simulink model "Ex5_3"  (R2016b)
settings: Solver=VariableStepAuto  StartTime=0.0  StopTime=runtime  RelTol=1e-3
values from neighbouring files (symbols this model uses):
  g = 9.81    [Ex5_3_init.m]
  i_smn0 = zeros(2,1)    [Ex5_3_init.m]
  J = 0.05    [Ex5_2_init.m]    (also in Ex5_3_init.m; Home54_init.m = 0.5; homepart51.m)
  Kd = 1    [Ex5_3_init.m]
  Ki = 1    [Ex5_3_init.m]
  Kp = 120    [Ex5_3_init.m]
  L_s = 0.085    [Ex5_2_init.m]    (also in Ex5_3_init.m; Home54_init.m)
  m = 40    [Ex5_3_init.m]
  p = 1    [Ex5_2_init.m]    (also in Ex5_3_init.m; Home54_init.m; homepart51.m)
  psi_Rmn0 = zeros(2,1)    [Ex5_3_init.m]
  r = 0.1    [Ex5_3_init.m]
  sigma = 1 - M^2/(L_s*L_r)    (= 0.0693425605536)    [Ex5_2_init.m]    (also in Ex5_3_init.m = 0.0693; Home54_init.m = 0.0693; homepart51.m)
  tau_r = 0.283    [Ex5_3_init.m]    (also in Home54_init.m)
  tau_sigma = 0.0102    [Ex5_3_init.m]
  U0 = 22    [Ex5_3_init.m]
  Us = sqrt(2)*Uphase    [Ex5_2_init.m]    (also in Ex5_3_init.m = Us_rat/Ws_rat * ws)
  Us_rat = Us    [Ex5_3_init.m]
  Wk = 50*2*pi    (= 314.159265359)    [Ex5_3_init.m]
  ws = 50*2*pi    (= 314.159265359)    [Ex5_2_init.m]    (also in Ex5_3_init.m)
  Ws_rat = 50*2*pi    (= 314.159265359)    [Ex5_3_init.m]
  Wslip_max = 49    [Ex5_3_init.m]
undefined symbols (not defined in the file or in its folder): sigbuilder_block
settings Model: Creator=Niels  LastModifiedBy=Niels

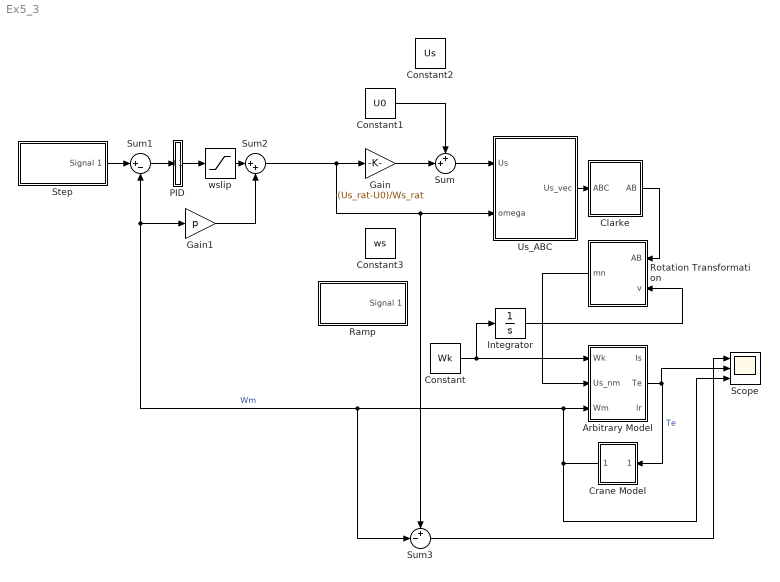
== system Ex5_3 ==
  Arbitrary Model : Subsystem
  Clarke : Subsystem
  Constant : Constant  Value=Wk
  Constant1 : Constant  Value=U0
  Constant2 : Constant  Value=Us
  Constant3 : Constant  Value=ws
  Crane Model : Subsystem
  Gain : Gain  Gain=(Us_rat-U0)/Ws_rat
  Gain1 : Gain  Gain=p
  Integrator : Integrator
  PID : Subsystem
  Ramp : Subsystem  Tag=STV Subsys  LoadFcn=sigbuilder_block('load');  StartFcn=sigbuilder_block('start');  StopFcn=sigbuilder_block('stop');  ClipboardFcn=sigbuilder_block('clipboard');  mask(Sigbuilder block){tuvar=[0:10]}
      mask help: Simulink:masks:SigbuilderBlock_MD
      mask init:
      | if ~strcmp(get_param(bdroot(gcbh),'SimulationStatus'),'stopped') tuvar = sigbuilder_block('maskInit'); end
      settings: CopyFcn=sigbuilder_block('copy');  DeleteFcn=sigbuilder_block('delete');  ModelCloseFcn=sigbuilder_block('modelClose');  PreSaveFcn=sigbuilder_block('preSave');  PauseFcn=sigbuilder_block('pause');  ContinueFcn=sigbuilder_block('continue');  NameChangeFcn=sigbuilder_block('namechange');  OpenFcn=sigbuilder_block('open',[437.6 199.2 550.4 400 ]);  CloseFcn=sigbuilder_block('close');
      mask Display: plot(0, 0, 100, 100,[2, 2, 32, 32, 2], [68, 8, 8, 68, 68],[32, 2], [38, 38], [32, 19, 2],[53, 60, 44], [32, 17, 17, 2],[16, 16, 31, 31]);txt = getActiveGroup(gcbh);text(2, 100, txt,'verticalAlignment', 'top');
  "Rotation Transformation " : Subsystem
  Scope : Scope  NumInputPorts=3
  Step : Subsystem  Tag=STV Subsys  LoadFcn=sigbuilder_block('load');  StartFcn=sigbuilder_block('start');  StopFcn=sigbuilder_block('stop');  ClipboardFcn=sigbuilder_block('clipboard');  mask(Sigbuilder block){tuvar=[0:10]}
      mask help: Simulink:masks:SigbuilderBlock_MD
      mask init:
      | if ~strcmp(get_param(bdroot(gcbh),'SimulationStatus'),'stopped') tuvar = sigbuilder_block('maskInit'); end
      settings: CopyFcn=sigbuilder_block('copy');  DeleteFcn=sigbuilder_block('delete');  ModelCloseFcn=sigbuilder_block('modelClose');  PreSaveFcn=sigbuilder_block('preSave');  PauseFcn=sigbuilder_block('pause');  ContinueFcn=sigbuilder_block('continue');  NameChangeFcn=sigbuilder_block('namechange');  OpenFcn=sigbuilder_block('open',[437.6 199.2 550.4 400 ]);  CloseFcn=sigbuilder_block('close');
      mask Display: plot(0, 0, 100, 100,[2, 2, 32, 32, 2], [68, 8, 8, 68, 68],[32, 2], [38, 38], [32, 19, 2],[53, 60, 44], [32, 17, 17, 2],[16, 16, 31, 31]);txt = getActiveGroup(gcbh);text(2, 100, txt,'verticalAlignment', 'top');
  Sum : Sum  Inputs=++|
  Sum1 : Sum  Inputs=|+-
  Sum2 : Sum  Inputs=|++
  Sum3 : Sum  Inputs=+-|
  Us_ABC : Subsystem
  wslip : Saturate  UpperLimit=Wslip_max  LowerLimit=-Wslip_max
  wires:
  Us_ABC/1(Us_vec) -> Clarke/1(ABC)
  Arbitrary Model/2(Te) -> Scope/2, Crane Model/1(Te)  "Te"
  Crane Model/1(wm) -> Scope/3, Arbitrary Model/3(Wm), Sum3/2, Gain1/1, Sum1/2  "Wm"
  Clarke/1(AB) -> "Rotation Transformation "/1(AB)
  "Rotation Transformation "/1(mn) -> Arbitrary Model/2(Us_nm)
  Integrator/1 -> "Rotation Transformation "/2(v)
  Gain/1 -> Sum/2
  Constant1/1 -> Sum/1
  Constant/1 -> Arbitrary Model/1(Wk), Integrator/1
  Step/1(Signal 1) -> Sum1/1
  Sum1/1 -> PID/1(In1)
  wslip/1 -> Sum2/1
  Sum2/1 -> Us_ABC/2(omega), Sum3/1, Gain/1
  Gain1/1 -> Sum2/2
  PID/1(Out1) -> wslip/1
  Sum3/1 -> Scope/1
  Sum/1 -> Us_ABC/1(Us)

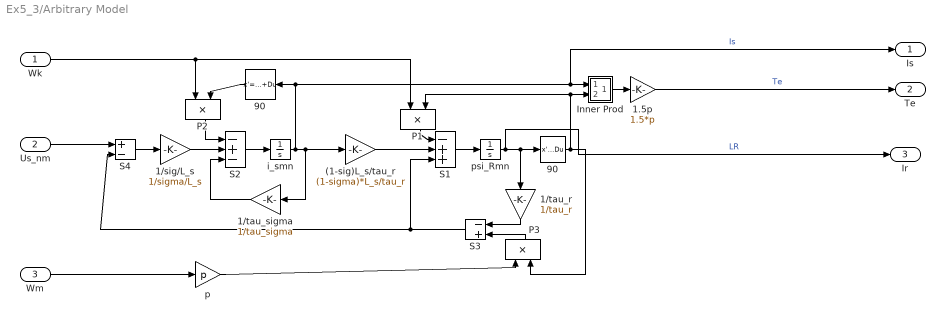
== system Ex5_3/Arbitrary Model ==
  Wk : Inport
  Us_nm : Inport  Port=2
  Wm : Inport  Port=3
  (1-sig)L_s/tau_r : Gain  Gain=(1-sigma)*L_s/tau_r  SaturateOnIntegerOverflow=on  OutDataTypeStr=Inherit: Same as input  ParamDataTypeStr=Inherit: Same as input
  1.5p : Gain  Gain=1.5*p  SaturateOnIntegerOverflow=on  OutDataTypeStr=Inherit: Same as input  ParamDataTypeStr=Inherit: Same as input
  1/sig/L_s : Gain  Gain=1/sigma/L_s  SaturateOnIntegerOverflow=on  OutDataTypeStr=Inherit: Same as input  ParamDataTypeStr=Inherit: Same as input
  1/tau_r : Gain  Gain=1/tau_r  SaturateOnIntegerOverflow=on  OutDataTypeStr=Inherit: Same as input  ParamDataTypeStr=Inherit: Same as input
  1/tau_sigma : Gain  Gain=1/tau_sigma  SaturateOnIntegerOverflow=on  OutDataTypeStr=Inherit: Same as input  ParamDataTypeStr=Inherit: Same as input
  90 : StateSpace  A=[]  B=[]  C=[]  D=K  X0=0  mask(Matrix gain){K=[0 -1;1 0]}
      mask prompts: K "Gain matrix:"
      mask help: Matrix Gain.
      mask Help: Multiplies input vector by entered matrix to produce output vector (y=Au).
      mask Display: disp('K')
  "90 " : StateSpace  A=[]  B=[]  C=[]  D=K  X0=0  mask(Matrix gain){K=[0 -1;1 0]}
      mask prompts: K "Gain matrix:"
      mask help: Matrix Gain.
      mask Help: Multiplies input vector by entered matrix to produce output vector (y=Au).
      mask Display: disp('K')
  Inner Prod : Subsystem  mask(Dot Product){}
      mask help:
      | Inner (dot) product.
      | y=sum(u1.*u2)
      mask Help: Computes the inner (dot) product of the inputs: sum(u1.*u2).  The inputs are vectors of the same length. Output is a scalar.
      mask Display: disp('.\n')
  P1 : Product  SaturateOnIntegerOverflow=on  RndMeth=Zero  InputSameDT=on  OutDataTypeStr=Inherit: Same as first input
  P2 : Product  SaturateOnIntegerOverflow=on  RndMeth=Zero  InputSameDT=on  OutDataTypeStr=Inherit: Same as first input
  P3 : Product  SaturateOnIntegerOverflow=on  RndMeth=Zero  InputSameDT=on  OutDataTypeStr=Inherit: Same as first input
  S1 : Sum  Inputs=-++  SaturateOnIntegerOverflow=on  InputSameDT=on  OutDataTypeStr=Inherit: Same as first input
  S2 : Sum  Inputs=-+-  SaturateOnIntegerOverflow=on  InputSameDT=on  OutDataTypeStr=Inherit: Same as first input
  S3 : Sum  Inputs=-+  SaturateOnIntegerOverflow=on  InputSameDT=on  OutDataTypeStr=Inherit: Same as first input
  S4 : Sum  Inputs=+-  SaturateOnIntegerOverflow=on  InputSameDT=on  OutDataTypeStr=Inherit: Same as first input
  i_smn : Integrator  InitialCondition=i_smn0
  "p " : Gain  Gain=p  SaturateOnIntegerOverflow=on  OutDataTypeStr=Inherit: Same as input  ParamDataTypeStr=Inherit: Same as input
  psi_Rmn : Integrator  InitialCondition=psi_Rmn0
  Is : Outport
  Te : Outport  Port=2
  Ir : Outport  Port=3
  wires:
  P2/1 -> S2/1
  Wm/1 -> "p "/1
  S4/1 -> 1/sig/L_s/1
  "p "/1 -> P3/1
  "90 "/1 -> P3/2, Inner Prod/2(in_2), P1/2
  S3/1 -> S1/3, S4/2
  S2/1 -> i_smn/1
  1/tau_sigma/1 -> S2/3
  P1/1 -> S1/1
  (1-sig)L_s/tau_r/1 -> S1/2
  1.5p/1 -> Te/1  "Te"
  Us_nm/1 -> S4/1
  1/tau_r/1 -> S3/1
  S1/1 -> psi_Rmn/1
  Inner Prod/1(out_1) -> 1.5p/1
  psi_Rmn/1 -> Ir/1, "90 "/1, 1/tau_r/1  "LR"
  P3/1 -> S3/2
  Wk/1 -> P1/1, P2/1
  90/1 -> P2/2
  i_smn/1 -> (1-sig)L_s/tau_r/1, 1/tau_sigma/1, 90/1, Is/1, Inner Prod/1(in_1)  "Is"
  1/sig/L_s/1 -> S2/2

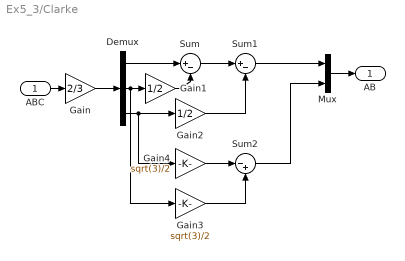
== system Ex5_3/Clarke ==
  ABC : Inport
  Demux : Demux  Outputs=3
  Gain : Gain  Gain=2/3
  Gain1 : Gain  Gain=1/2
  Gain2 : Gain  Gain=1/2
  Gain3 : Gain  Gain=sqrt(3)/2
  Gain4 : Gain  Gain=sqrt(3)/2
  Mux : Mux  Inputs=2
  Sum : Sum  Inputs=|+-
  Sum1 : Sum  Inputs=|+-
  Sum2 : Sum  Inputs=|-+
  AB : Outport
  wires:
  ABC/1 -> Gain/1
  Mux/1 -> AB/1
  Gain/1 -> Demux/1
  Demux/1 -> Sum/1
  Demux/2 -> Gain3/1, Gain1/1
  Gain1/1 -> Sum/2
  Sum/1 -> Sum1/1
  Sum1/1 -> Mux/1
  Demux/3 -> Gain4/1, Gain2/1
  Gain2/1 -> Sum1/2
  Gain4/1 -> Sum2/1
  Gain3/1 -> Sum2/2
  Sum2/1 -> Mux/2

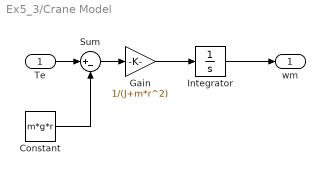
== system Ex5_3/Crane Model ==
  Te : Inport
  Constant : Constant  Value=m*g*r
  Gain : Gain  Gain=1/(J+m*r^2)
  Integrator : Integrator
  Sum : Sum  Inputs=|+-
  wm : Outport
  wires:
  Gain/1 -> Integrator/1
  Integrator/1 -> wm/1
  Te/1 -> Sum/1
  Sum/1 -> Gain/1
  Constant/1 -> Sum/2

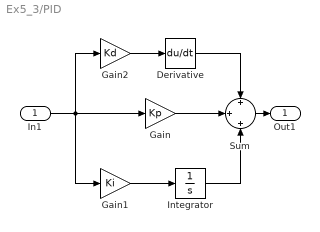
== system Ex5_3/PID ==
  In1 : Inport
  Derivative : Derivative
  Gain : Gain  Gain=Kp
  Gain1 : Gain  Gain=Ki
  Gain2 : Gain  Gain=Kd
  Integrator : Integrator
  Sum : Sum  Inputs=+|+|+
  Out1 : Outport
  wires:
  In1/1 -> Gain2/1, Gain1/1, Gain/1
  Gain1/1 -> Integrator/1
  Sum/1 -> Out1/1
  Gain/1 -> Sum/2
  Integrator/1 -> Sum/3
  Gain2/1 -> Derivative/1
  Derivative/1 -> Sum/1

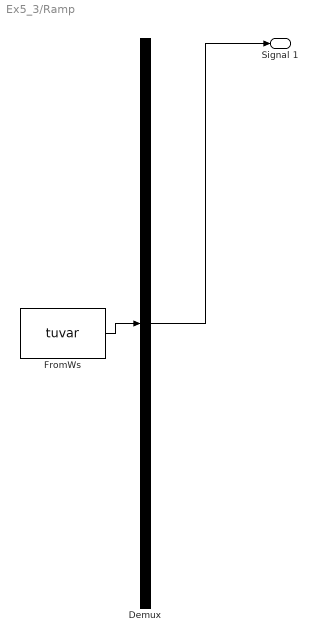
== system Ex5_3/Ramp ==
  Demux : Demux  Tag=STV Demux  Outputs=1
  FromWs : FromWorkspace  Tag=STV FromWs  VariableName=tuvar  SampleTime=0
      SigBuilderData=|
      | common.afterFinalStr = 'Extrapolate'
      | common.sampleTime = 0
      | dataSet.timeRange = [0 100]
      | dataSet.name = 'Group 1'
      | sbobj.Groups.Name = 'Group 1'
      | sbobj.Groups.Signals.Name = 'Signal 1'
      | sbobj.Groups.Signals.XData = [0 3 100]
      | sbobj.Groups.Signals.YData = [56.5486677646 314.159265359 314.159265359]
      | sbobj.Groups.TimeRange = [0 100]
  Signal 1 : Outport  Tag=STV Outport
  wires:
  Demux/1 -> Signal 1/1
  FromWs/1 -> Demux/1

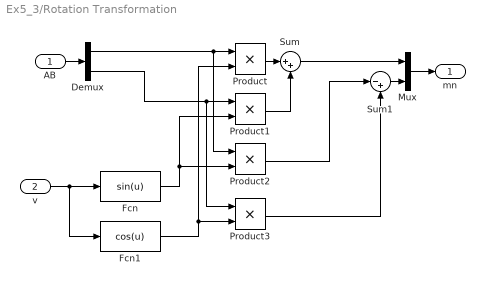
== system Ex5_3/Rotation Transformation  ==
  AB : Inport
  v : Inport  Port=2
  Demux : Demux  Outputs=2
  Fcn : Fcn  Expr=sin(u)
  Fcn1 : Fcn  Expr=cos(u)
  Mux : Mux  Inputs=2
  Product{,1..3} (4 alike) : Product
  Sum : Sum  Inputs=|++
  Sum1 : Sum  Inputs=|-+
  mn : Outport
  wires:
  v/1 -> Fcn1/1, Fcn/1
  Mux/1 -> mn/1
  AB/1 -> Demux/1
  Sum/1 -> Mux/1
  Product/1 -> Sum/1
  Demux/1 -> Product2/1, Product/1
  Fcn1/1 -> Product3/2, Product/2
  Demux/2 -> Product3/1, Product1/1
  Fcn/1 -> Product2/2, Product1/2
  Product1/1 -> Sum/2
  Sum1/1 -> Mux/2
  Product2/1 -> Sum1/1
  Product3/1 -> Sum1/2

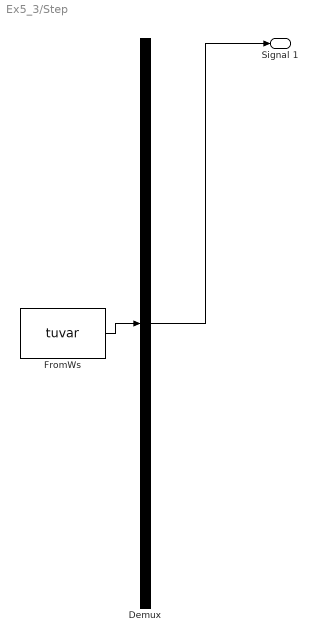
== system Ex5_3/Step ==
  Demux : Demux  Tag=STV Demux  Outputs=1
  FromWs : FromWorkspace  Tag=STV FromWs  VariableName=tuvar  SampleTime=0
      SigBuilderData=|
      | common.afterFinalStr = 'Extrapolate'
      | common.sampleTime = 0
      | dataSet.timeRange = [0 10]
      | dataSet.name = 'Group 1'
      | sbobj.Groups.Name = 'Group 1'
      | sbobj.Groups.Signals.Name = 'Signal 1'
      | sbobj.Groups.Signals.XData = [0 10]
      | sbobj.Groups.Signals.YData = [314.159265359 314.159265359]
  Signal 1 : Outport  Tag=STV Outport
  wires:
  Demux/1 -> Signal 1/1
  FromWs/1 -> Demux/1

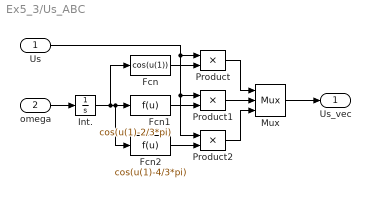
== system Ex5_3/Us_ABC ==
  Us : Inport
  omega : Inport  Port=2
  Fcn : Fcn  Expr=cos(u(1))
  Fcn1 : Fcn  Expr=cos(u(1)-2/3*pi)
  Fcn2 : Fcn  Expr=cos(u(1)-4/3*pi)
  Int. : Integrator
  Mux : Mux  Inputs=3
  Product : Product  SaturateOnIntegerOverflow=on  RndMeth=Zero  InputSameDT=on  OutDataTypeStr=Inherit: Same as first input
  Product1 : Product  SaturateOnIntegerOverflow=on  RndMeth=Zero  InputSameDT=on  OutDataTypeStr=Inherit: Same as first input
  Product2 : Product  SaturateOnIntegerOverflow=on  RndMeth=Zero  InputSameDT=on  OutDataTypeStr=Inherit: Same as first input
  Us_vec : Outport
  wires:
  Fcn2/1 -> Product2/2
  Fcn1/1 -> Product1/2
  Product/1 -> Mux/1
  Product2/1 -> Mux/3
  Mux/1 -> Us_vec/1
  Product1/1 -> Mux/2
  omega/1 -> Int./1
  Us/1 -> Product/1, Product1/1, Product2/1
  Fcn/1 -> Product/2
  Int./1 -> Fcn1/1, Fcn2/1, Fcn/1

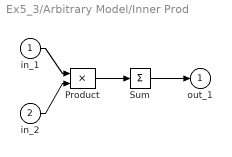
== system Ex5_3/Arbitrary Model/Inner Prod ==
  in_1 : Inport
  in_2 : Inport  Port=2
  Product : Product  SaturateOnIntegerOverflow=on  RndMeth=Zero  InputSameDT=on  OutDataTypeStr=Inherit: Same as first input
  Sum : Sum  Inputs=+  SaturateOnIntegerOverflow=on  InputSameDT=on  OutDataTypeStr=Inherit: Same as first input
  out_1 : Outport
  wires:
  in_2/1 -> Product/2
  in_1/1 -> Product/1
  Product/1 -> Sum/1
  Sum/1 -> out_1/1
